simulink model "penddemo"  (Simulink 7.6)
settings: Solver=ode45  SolverMode=SingleTasking  StartTime=0  StopTime=inf  MaxStep=0.02  RelTol=1e-3  AbsTol=1e-6
undefined symbols (not defined in the file or in its folder): K, Ts
Description:
  | Inverted Pendulum with Animation
  | 
  | The animation is created using MATLAB(R) Handle Graphics(R).  The animation block is a masked
  | S-function.  For more information, use the context menu to look under the Animation block's mask
  | and open the S-function for editing.
settings Model: Creator=The MathWorks Inc.  ExtModeAutoUpdateStatusClock=off
settings DataIOCC: ExternalInput=[]  InitialState=[]  LimitDataPoints=off  SaveOutput=off  SaveTime=off
settings OptimizationCC: BlockReduction=off  BooleanDataType=off  InitFltsAndDblsToZero=on
settings DebuggingCC: SaveWithParameterizedLinksMsg=none  SignalResolutionControl=TryResolveAllWithWarning  SolverPrmCheckMsg=none  MultiTaskDSMMsg=warning  MultiTaskCondExecSysMsg=none  SigSpecEnsureSampleTimeMsg=none
settings HardwareCC: TargetUnknown=on
settings RTWCC: IncludeERTFirstTime=on
settings GRTTargetCC: TargetFcnLib=ansi_tfl_tmw.mat

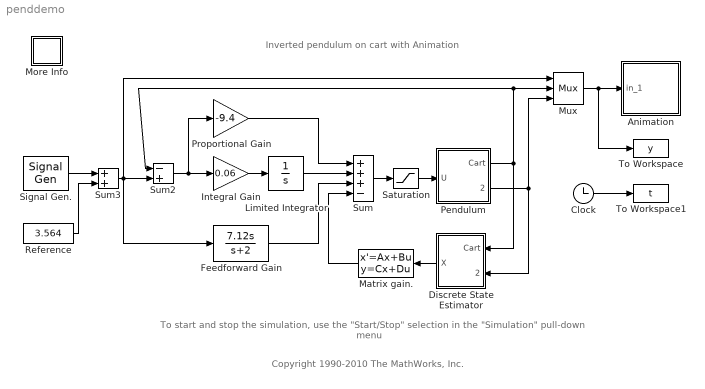
== system penddemo ==
  note: Inverted pendulum on cart with Animation
  note: To start and stop the simulation, use the "Start/Stop"
      | selection in the "Simulation" pull-down menu
  note: Copyright 1990-2010 The MathWorks, Inc.
  Animation : Subsystem  mask(Pendulum plot){RefBlock=Reference}
      mask prompts: RefBlock "DC reference signal block name:"
      mask help: Pendulum plot
      mask Help: Pendulum animation function using Handle graphics.
      mask Display: plot([-10 10],[0 0],[-2 -2 2 2],[0 1 1 0],[0 3],[1 5])
  Clock : Clock
      settings: Decimation=10
  Discrete State Estimator : Subsystem  mask(Pendulum Discrete state estimator){Ts =0.02}
      mask prompts: Ts  "Sample time"
      mask help: Pendulum discrete state estimator
      mask Help: The states of the pendulum and cart system are the pendulum angle and angular velocity and cart position and velocity.  Since the sensors output the pendulum angle and cart position, this state estimator just does a one step difference calculation to get the velocities.
  Feedforward Gain : TransferFcn  Numerator=[7.12 0]  Denominator=[1 2]
  Integral Gain : Gain  Gain=0.06  SaturateOnIntegerOverflow=on  OutDataTypeStr=Inherit: Same as input  ParamDataTypeStr=Inherit: Same as input
  Limited Integrator : Integrator  LimitOutput=on  UpperSaturationLimit=5  LowerSaturationLimit=-5
  Matrix gain. : StateSpace  A=[]  B=[]  C=[]  D=K  mask(Matrix gain){K =[0 -18 -166.5 -15.2]}
      mask prompts: K  "Gain matrix:"
      mask help: Matrix Gain:
      mask Help: Multiplies input vector by entered matrix to produce output vector.
      mask Display: disp('LQR')
  More Info : Subsystem
      settings: OpenFcn=showdemo(bdroot(gcb))
      mask Display: disp('?')
  Mux : Mux  Inputs=3
  Pendulum : Subsystem  mask(Inverted pendulum on cart){Mcart=0.455, m=0.21, l=0.61/2, g=9.8}
      mask prompts: Mcart "Mass of cart (kg):"; m "Mass of pendulum (kg):"; l "Distance to pendulum center of mass(m):"; g "Acceleration of gravity (m/s^2):"
      mask help: Unmask and double-click to see dynamics
      mask Help: Nonlinear dynamics of inverted pendulum on cart.
  Proportional Gain : Gain  Gain=-9.4  SaturateOnIntegerOverflow=on  OutDataTypeStr=Inherit: Same as input  ParamDataTypeStr=Inherit: Same as input
  Reference : Constant  Value=3.564
  Saturation : Saturate  UpperLimit=10  LowerLimit=-10
  Signal Gen. : SignalGenerator  WaveForm=square  Amplitude=0.000000  Frequency=0.400000  Units=rad/sec
  Sum : Sum  Inputs=+++-  SaturateOnIntegerOverflow=on  InputSameDT=on  OutDataTypeStr=Inherit: Same as first input
  Sum2 : Sum  Inputs=-+  SaturateOnIntegerOverflow=on  InputSameDT=on  OutDataTypeStr=Inherit: Same as first input
  Sum3 : Sum  SaturateOnIntegerOverflow=on  InputSameDT=on  OutDataTypeStr=Inherit: Same as first input
  To Workspace : ToWorkspace  VariableName=y  SampleTime=0.1  SaveFormat=Array
  To Workspace1 : ToWorkspace  VariableName=t  SampleTime=0.1  SaveFormat=Array
  wires:
  Sum2/1 -> Proportional Gain/1, Integral Gain/1
  Discrete State Estimator/1(X) -> Matrix gain./1
  Mux/1 -> To Workspace/1, Animation/1(in_1)
  Pendulum/2(Pendulum) -> Mux/3, Discrete State Estimator/2(Pendulum)
  Sum3/1 -> Mux/1, Feedforward Gain/1, Sum2/2
  Integral Gain/1 -> Limited Integrator/1
  Sum/1 -> Saturation/1
  Proportional Gain/1 -> Sum/1
  Feedforward Gain/1 -> Sum/3
  Reference/1 -> Sum3/2
  Signal Gen./1 -> Sum3/1
  Matrix gain./1 -> Sum/4
  Limited Integrator/1 -> Sum/2
  Pendulum/1(Cart) -> Sum2/1, Mux/2, Discrete State Estimator/1(Cart)
  Saturation/1 -> Pendulum/1(U)
  Clock/1 -> To Workspace1/1

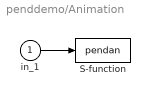
== system penddemo/Animation ==
  in_1 : Inport
  S-function : S-Function  FunctionName=pendan  Parameters=RefBlock  EnableBusSupport=off
      settings: DeleteFcn=pendan([],[],[],'DeleteBlock');
  wires:
  in_1/1 -> S-function/1

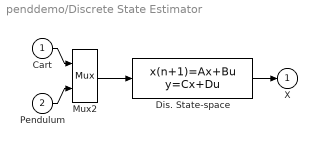
== system penddemo/Discrete State Estimator ==
  Cart : Inport
  Pendulum : Inport  Port=2
  Dis. State-space : DiscreteStateSpace  A=zeros(2)  B=-eye(2)/Ts  C=[0 0; 1 0; 0 0; 0 1]  D=[1 0; 1/Ts 0; 0 1; 0 1/Ts]  SampleTime=Ts
  Mux2 : Mux  Inputs=2
  X : Outport  InitialOutput=0
  wires:
  Pendulum/1 -> Mux2/2
  Dis. State-space/1 -> X/1
  Cart/1 -> Mux2/1
  Mux2/1 -> Dis. State-space/1

== system penddemo/More Info ==

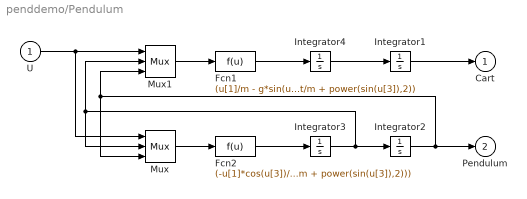
== system penddemo/Pendulum ==
  U : Inport
  Fcn1 : Fcn  Expr=(u[1]/m - g*sin(u[3])*cos(u[3]) + l*power(u[2],2)*sin(u[3]))/(Mcart/m + power(sin(u[3]),2))
  Fcn2 : Fcn  Expr=(-u[1]*cos(u[3])/m + (Mcart+m)*g*sin(u[3])/m - l*power(u[2],2)*sin(u[3])*cos(u[3]))/(l*(Mcart/m + power(sin(u[3]),2)))
  Integrator{1..4} (4 alike) : Integrator
  Mux : Mux  Inputs=3
  Mux1 : Mux  Inputs=3
  Cart : Outport  InitialOutput=0
  Pendulum : Outport  Port=2  InitialOutput=0
  wires:
  Integrator1/1 -> Cart/1
  Fcn2/1 -> Integrator3/1
  Mux/1 -> Fcn2/1
  Mux1/1 -> Fcn1/1
  Fcn1/1 -> Integrator4/1
  Integrator4/1 -> Integrator1/1
  U/1 -> Mux1/1, Mux/1
  Integrator3/1 -> Integrator2/1, Mux1/2, Mux/2
  Integrator2/1 -> Pendulum/1, Mux1/3, Mux/3
